simulink model "Arduino_STC"  (R2024b)
settings: Solver=FixedStepAuto  StartTime=0.0  StopTime=10.0  RelTol=1e-3  EnableMultiTasking=on
libraries: arduinolib x15
settings Model: ExtModeTrigDuration=2  Creator=chall  LastModifiedBy=chall
settings SolverCC: AutoInsertRateTranBlk=on
settings OptimizationCC: EnhancedBackFolding=on  PassReuseOutputArgsAs=Individual arguments  ZeroExternalMemoryAtStartup=off  ZeroInternalMemoryAtStartup=off  MaxStackSize=64  OptimizeBlockOrder=speed  DifferentSizesBufferReuse=on  OptimizationCustomize=off  EfficientTunableParamExpr=on
settings DebuggingCC: ParameterTunabilityLossMsg=error
settings HardwareCC: ProdBitPerInt=16  ProdBitPerPointer=16  ProdBitPerSizeT=16  ProdBitPerPtrDiffT=16  ProdLargestAtomicFloat=None  ProdWordSize=8  ProdHWDeviceType=Atmel->AVR  UseEmbeddedCoderFeatures=off  UseSimulinkCoderFeatures=off
settings SFSimCC: MATLABDynamicMemAlloc=off
settings RTWCC: Description=Embedded Coder  SystemTargetFile=ert.tlc  HardwareBoard=Arduino Uno  TemplateMakefile=ert_default_tmf  Toolchain=Arduino AVR  BuildConfiguration=Faster Runs
settings CodeAppCC: ForceParamTrailComments=on  IgnoreCustomStorageClasses=off  OperatorAnnotations=on  SimulinkDataObjDesc=on  SFDataObjDesc=on  InsertBlockDesc=on
settings ERTTargetCC: SupportContinuousTime=on  SupportNonInlinedSFcns=on  SupportVariableSizeSignals=on  ExtModeTransport=3  ExtModeStaticAlloc=on  ExtModeAutomaticAllocSize=off  ExtModeStaticAllocSize=250  ExtModeMexFile=ext_xcp  ExtModeIntrfLevel=Level2 - Open  InlinedParameterPlacement=Hierarchical

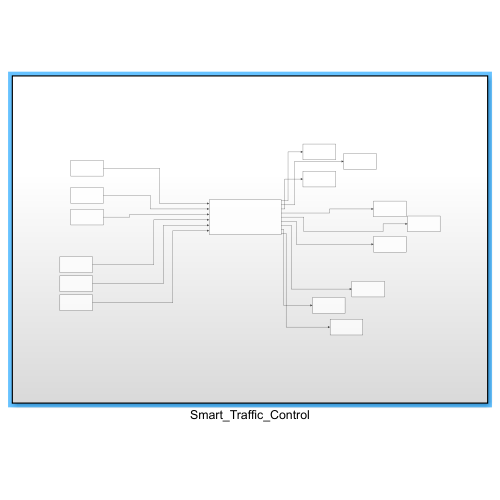
[thumbnail: Simulink's stored preview of the top-level diagram]
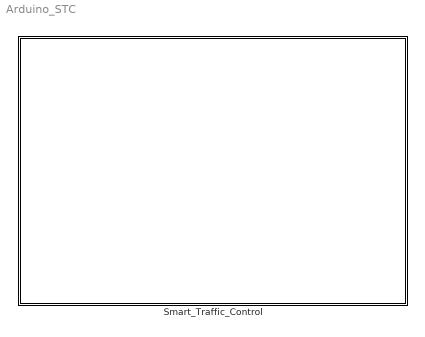
== system Arduino_STC ==
  Smart_Traffic_Control : Subsystem

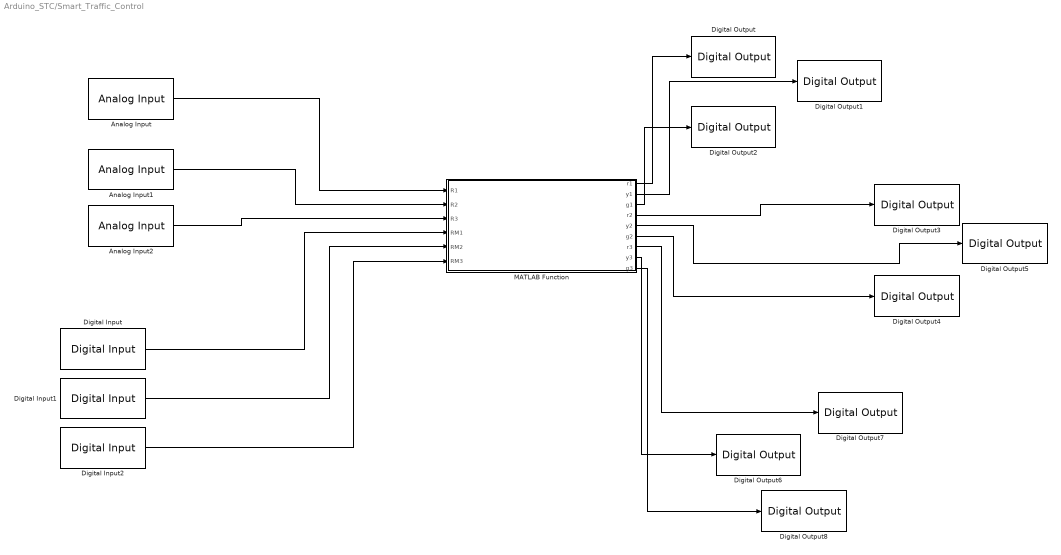
== system Arduino_STC/Smart_Traffic_Control ==
  Analog Input : arduinolib/Analog Input  pinNumber=0  ReadResultsOnly=off  ConversionTriggerSource=Software  ExternalTriggerType=uint32( 0 )  OutputDataType=uint16  EnableConversionCompleteNotify=off  EnableOuputStatus=off  SampleTime=-1  blockPlatform=arduino
      settings: SourceProductName=Common
  Analog Input1 : arduinolib/Analog Input  pinNumber=1  ReadResultsOnly=off  ConversionTriggerSource=Software  ExternalTriggerType=uint32( 0 )  OutputDataType=uint16  EnableConversionCompleteNotify=off  EnableOuputStatus=off  SampleTime=-1  blockPlatform=arduino
      settings: SourceProductName=Common
  Analog Input2 : arduinolib/Analog Input  pinNumber=2  ReadResultsOnly=off  ConversionTriggerSource=Software  ExternalTriggerType=uint32( 0 )  OutputDataType=uint16  EnableConversionCompleteNotify=off  EnableOuputStatus=off  SampleTime=-1  blockPlatform=arduino
      settings: SourceProductName=Common
  Digital Input : arduinolib/Digital Input  pinNumber=2  mode=Default  Direction=input  SampleTime=0.1  blockPlatform=arduino
      settings: SourceProductName=Common
  Digital Input1 : arduinolib/Digital Input  pinNumber=3  mode=Default  Direction=input  SampleTime=0.1  blockPlatform=arduino
      settings: SourceProductName=Common
  Digital Input2 : arduinolib/Digital Input  pinNumber=4  mode=Default  Direction=input  SampleTime=0.1  blockPlatform=arduino
      settings: SourceProductName=Common
  Digital Output : arduinolib/Digital Output  pinNumber=5  Direction=output  blockPlatform=arduino
      settings: SourceProductName=Common
  Digital Output1 : arduinolib/Digital Output  pinNumber=6  Direction=output  blockPlatform=arduino
      settings: SourceProductName=Common
  Digital Output2 : arduinolib/Digital Output  pinNumber=7  Direction=output  blockPlatform=arduino
      settings: SourceProductName=Common
  Digital Output3 : arduinolib/Digital Output  pinNumber=8  Direction=output  blockPlatform=arduino
      settings: SourceProductName=Common
  Digital Output4 : arduinolib/Digital Output  pinNumber=10  Direction=output  blockPlatform=arduino
      settings: SourceProductName=Common
  Digital Output5 : arduinolib/Digital Output  pinNumber=9  Direction=output  blockPlatform=arduino
      settings: SourceProductName=Common
  Digital Output6 : arduinolib/Digital Output  pinNumber=12  Direction=output  blockPlatform=arduino
      settings: SourceProductName=Common
  Digital Output7 : arduinolib/Digital Output  pinNumber=11  Direction=output  blockPlatform=arduino
      settings: SourceProductName=Common
  Digital Output8 : arduinolib/Digital Output  pinNumber=13  Direction=output  blockPlatform=arduino
      settings: SourceProductName=Common
  MATLAB Function : MATLAB Function  TreatAsAtomicUnit=on
  wires:
  MATLAB Function/8(y3) -> Digital Output6/1
  Digital Input2/1 -> MATLAB Function/6(RM3)
  MATLAB Function/7(r3) -> Digital Output7/1
  MATLAB Function/9(g3) -> Digital Output8/1
  MATLAB Function/4(r2) -> Digital Output3/1
  MATLAB Function/2(y1) -> Digital Output1/1
  MATLAB Function/5(y2) -> Digital Output5/1
  MATLAB Function/1(r1) -> Digital Output/1
  MATLAB Function/3(g1) -> Digital Output2/1
  MATLAB Function/6(g2) -> Digital Output4/1
  Analog Input1/1 -> MATLAB Function/2(R2)
  Analog Input/1 -> MATLAB Function/1(R1)
  Analog Input2/1 -> MATLAB Function/3(R3)
  Digital Input/1 -> MATLAB Function/4(RM1)
  Digital Input1/1 -> MATLAB Function/5(RM2)

== matlab function Arduino_STC/Smart_Traffic_Control/MATLAB Function ==
  data: R1 input; r1 output; R2 input; R3 input; RM1 input; RM2 input; RM3 input; y1 output; g1 output; r2 output; y2 output; g2 output; r3 output; y3 output; g3 output
function [r1,y1,g1,r2,y2,g2,r3,y3,g3] = fcn(R1,R2,R3,RM1,RM2,RM3)


r1 = 0; y1 = 0; g1 = 0;
r2 = 0; y2 = 0; g2 = 0;
r3 = 0; y3 = 0; g3 = 0;


   if R1 > R2 && R1 > R3
        r1 = 0; y1 = 0; g1 = 1;
        r2 = 1; y2 = 0; g2 = 0;
        r3 = 0; y3 = 1; g3 = 0;
    elseif R2 > R3 && R2>R1
        r1 = 0; y1 = 1; g1 = 0;
        r2 = 0; y2 = 0; g2 = 1;
        r3 = 1; y3 = 0; g3 = 0;
    elseif R3 > R1 && R3 > R2
        r1 = 1; y1 = 0; g1 = 0;
        r2 = 0; y2 = 1; g2 = 0;
        r3 = 0; y3 = 0; g3 = 1;
   end

    if RM1 == 1
        r1 = 0; y1 = 0; g1 = 1;
        r2 = 1; y2 = 0; g2 = 0;
        r3 = 0; y3 = 1; g3 = 0;
    elseif RM2 == 1  
        r1 = 0; y1 = 1; g1 = 0;
        r2 = 0; y2 = 0; g2 = 1;
        r3 = 1; y3 = 0; g3 = 0;
    elseif RM3 == 1
        r1 = 1; y1 = 0; g1 = 0;
        r2 = 0; y2 = 1; g2 = 0;
        r3 = 0; y3 = 0; g3 = 1;
   
   
end



end
